simulink model "predict_RUL_with_ML"  (R2022a)
settings: Solver=FixedStepDiscrete  StartTime=0.0  StopTime=10.0  FixedStep=1  RelTol=1e-3
libraries: simulink x1, statsLibrary x1
settings Model: Creator=tshintai  LastModifiedBy=tshintai
settings OptimizationCC: DefaultParameterBehavior=Inlined  EnhancedBackFolding=on  PassReuseOutputArgsAs=Individual arguments  ZeroExternalMemoryAtStartup=off  ZeroInternalMemoryAtStartup=off  OptimizeBlockOrder=speed  DifferentSizesBufferReuse=on  OptimizationCustomize=off  EfficientTunableParamExpr=on
settings DebuggingCC: ParameterTunabilityLossMsg=error  UnconnectedInputMsg=warning  UnconnectedOutputMsg=warning  UnconnectedLineMsg=warning
settings SFSimCC: MATLABDynamicMemAlloc=off
settings RTWCC: SystemTargetFile=ert.tlc  TemplateMakefile=ert_default_tmf  GenerateReport=on  LaunchReport=on  GenerateCodeMetricsReport=on  DLArmComputeVersion=19.05
settings CodeAppCC: ForceParamTrailComments=on  IgnoreCustomStorageClasses=off  MaxIdLength=256  OperatorAnnotations=on  SimulinkDataObjDesc=on  SFDataObjDesc=on  InsertBlockDesc=on
settings ERTTargetCC: TargetLangStandard=C99 (ISO)  GenerateSampleERTMain=on  SupportVariableSizeSignals=on  InlinedParameterPlacement=NonHierarchical  ERTCustomFileTemplate=example_file_process.tlc

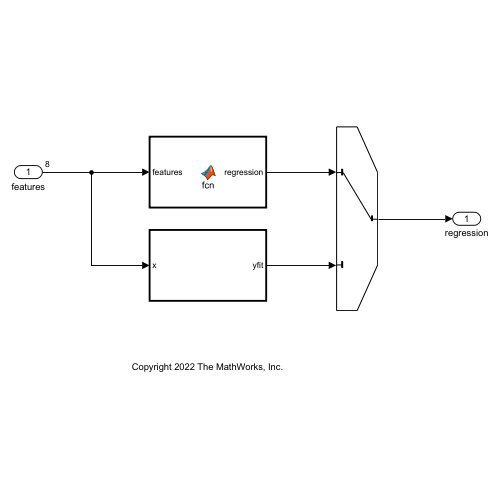
[thumbnail: Simulink's stored preview of the top-level diagram]
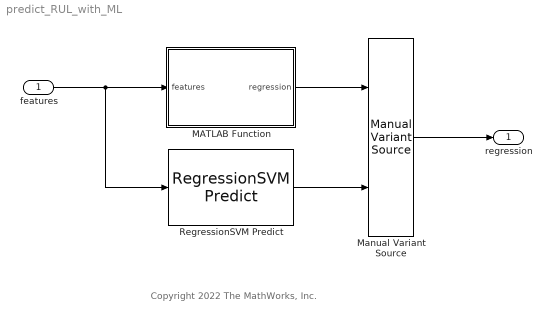
== system predict_RUL_with_ML ==
  note: Copyright 2022 The MathWorks, Inc.
  features : Inport  PortDimensions=8
  MATLAB Function : MATLAB Function  TreatAsAtomicUnit=on
  Manual Variant Source : simulink/Signal Routing/Manual Variant Source  NumChoices=2  LabelModeActiveChoice=V_1
  RegressionSVM Predict : statsLibrary/Regression/RegressionSVM Predict  TrainedLearner=trainedModel_SVM.RegressionSVM  OutMin=[]  OutMax=[]  KernelDataTypeStr=double  KernelOutMin=[]  KernelOutMax=[]
      settings: SourceProductBaseCode=ST
  regression : Outport
  wires:
  features/1 -> RegressionSVM Predict/1, MATLAB Function/1(features)
  MATLAB Function/1(regression) -> Manual Variant Source/1
  RegressionSVM Predict/1 -> Manual Variant Source/2
  Manual Variant Source/1 -> regression/1

== matlab function predict_RUL_with_ML/MATLAB Function ==
  data: features input; regression output
function regression = fcn(features)

% 列ベクトルが来た時は行ベクトルにする
if (size(features, 1) > 1)
    f_t = features';
else
    f_t = features;
end

regModel = loadLearnerForCoder('trainedModel.mat');

regression = predict(regModel, f_t);

end
